simulink model "CurrentSensorOffsetCalibrationComponent"  (R2025b)
settings: Solver=FixedStepDiscrete  StartTime=0.0  StopTime=10.0  RelTol=1e-3
settings Model: DataDictionary=TractionEmotorSoftwareArchInterfaceData.sldd  Creator=dakaihu  LastModifiedBy=dakaihu
settings OptimizationCC: ReuseModelBlockBuffer=off
settings RTWCC: GPUComputeCapability=3.5

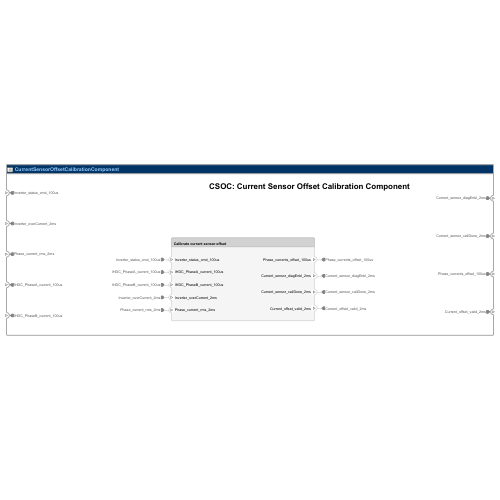
[thumbnail: Simulink's stored preview of the top-level diagram]
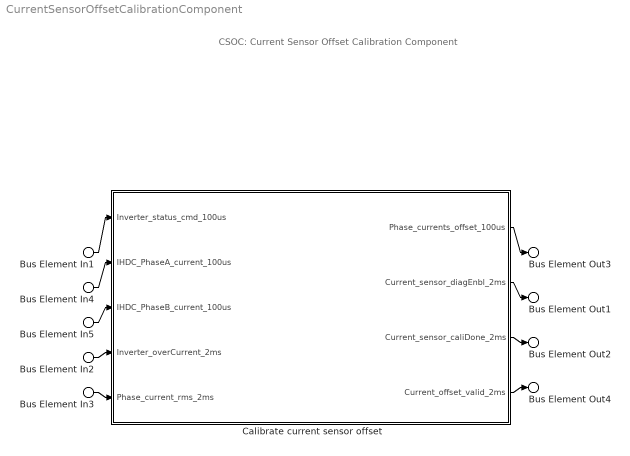
== system CurrentSensorOffsetCalibrationComponent ==
  note: CSOC: Current Sensor Offset Calibration Component
  Bus Element In1 : Inport  PortName=Inverter_status_cmd_100us
  Bus Element In2 : Inport  Port=2  PortName=Inverter_overCurrent_2ms
  Bus Element In3 : Inport  Port=3  PortName=Phase_current_rms_2ms
  Bus Element In4 : Inport  Port=4  PortName=IHDC_PhaseA_current_100us
  Bus Element In5 : Inport  Port=5  PortName=IHDC_PhaseB_current_100us
  Calibrate current sensor offset : Subsystem
      settings: PortSchema="{\"entries\":[{\"content\":{\"headerSize\":26,\"margin\":15,\"minimumSpacing\":25,\"sides\":[{\"content\":{\"connectorIds\":[\"In1\",\"In2\",\"In3\",\"In4\",\"In5\"]},\"type\":\"ConnectorPlacement.EquallySpacedRectSide\",\"uuid\":\"a0c63ab2-75fe-4bec-b2b0-6e2e00a1a5a4\"},{\"content\":{\"connectorIds\":[\"Out1\",\"Out2\",\"Out3\",\"Out4\"],\"side\":\"RIGHT\"},\"type\":\"ConnectorPlacement.EquallySpacedRectSide\",\"uuid\":\"05d605ea-8968-4533-a01c-bf4aae5caa93\"},{\"content\":{\"connectorIds\":[],\"side\":\"TOP\"},\"type\":\"ConnectorPlacement.EquallySpacedRectSide\",\"uuid\":\"27167c69-3967-4107-acce-f317c3d854af\"}]},\"type\":\"ConnectorPlacement.EquallySpacedConnector\",\"uuid\":\"c4d90da2-0f2a-4c00-bd24-85fead00d18f\"}],\"packageUris\":[\"http://schema.mathworks.com/mf0/Connector/R2020b\"],\"version\":\"1.0\"}"
  Bus Element Out1 : Outport  PortName=Current_sensor_diagEnbl_2ms
  Bus Element Out2 : Outport  Port=2  PortName=Current_sensor_caliDone_2ms
  Bus Element Out3 : Outport  Port=3  PortName=Phase_currents_offset_100us
  Bus Element Out4 : Outport  Port=4  PortName=Current_offset_valid_2ms
  wires:
  Bus Element In1/1 -> Calibrate current sensor offset/1(Inverter_status_cmd_100us)
  Bus Element In4/1 -> Calibrate current sensor offset/2(IHDC_PhaseA_current_100us)
  Bus Element In5/1 -> Calibrate current sensor offset/3(IHDC_PhaseB_current_100us)
  Bus Element In2/1 -> Calibrate current sensor offset/4(Inverter_overCurrent_2ms)
  Bus Element In3/1 -> Calibrate current sensor offset/5(Phase_current_rms_2ms)
  Calibrate current sensor offset/1(Phase_currents_offset_100us) -> Bus Element Out3/1
  Calibrate current sensor offset/2(Current_sensor_diagEnbl_2ms) -> Bus Element Out1/1
  Calibrate current sensor offset/3(Current_sensor_caliDone_2ms) -> Bus Element Out2/1
  Calibrate current sensor offset/4(Current_offset_valid_2ms) -> Bus Element Out4/1

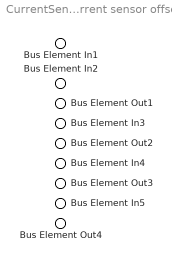
== system CurrentSensorOffsetCalibrationComponent/Calibrate current sensor offset ==
  Bus Element In1 : Inport  PortName=Inverter_status_cmd_100us
  Bus Element In2 : Inport  Port=2  PortName=IHDC_PhaseA_current_100us
  Bus Element In3 : Inport  Port=3  PortName=IHDC_PhaseB_current_100us
  Bus Element In4 : Inport  Port=4  PortName=Inverter_overCurrent_2ms
  Bus Element In5 : Inport  Port=5  PortName=Phase_current_rms_2ms
  Bus Element Out1 : Outport  PortName=Phase_currents_offset_100us
  Bus Element Out2 : Outport  Port=2  PortName=Current_sensor_diagEnbl_2ms
  Bus Element Out3 : Outport  Port=3  PortName=Current_sensor_caliDone_2ms
  Bus Element Out4 : Outport  Port=4  PortName=Current_offset_valid_2ms
